simulink model "Simulation"  (R2023b)
settings: Solver=FixedStepAuto  StartTime=0  StopTime=H  FixedStep=fixed_step_size  RelTol=1e-3
values from neighbouring files (symbols this model uses):
  a_p = load_pu(:,3)    [Matlab_1_Generate_Case_Params.m]
  a_q = load_pu(:,6)    [Matlab_1_Generate_Case_Params.m]
  b_p = load_pu(:,4)    [Matlab_1_Generate_Case_Params.m]
  b_q = load_pu(:,7)    [Matlab_1_Generate_Case_Params.m]
  Be = zeros(Nn,Ne)    [Matlab_1_Generate_Case_Params.m]
  Bibr = zeros(Nn,Nibr)    [Matlab_1_Generate_Case_Params.m]
  Bload = zeros(Nn,Nload)    [Matlab_1_Generate_Case_Params.m]
  Bsh = zeros(Nn,Nsh)    [Matlab_1_Generate_Case_Params.m]
  C_f = gen_pu(:,7)    [Matlab_1_Generate_Case_Params.m]
  c_p = load_pu(:,5)    [Matlab_1_Generate_Case_Params.m]
  c_q = load_pu(:,8)    [Matlab_1_Generate_Case_Params.m]
  C_sh = busC(busC~=0)    [Matlab_1_Generate_Case_Params.m]
  Cdc = gen_pu(:,3)    [Matlab_1_Generate_Case_Params.m]
  f_b = 50    [Matlab_1_Generate_Case_Params.m]
  fixed_step_size = 1e-4    (= 0.0001)    [Matlab_2_Ref_Loop.m]
  ix_ibr_max = gen_pu(:,9) .* s_ibr_nom    [Matlab_1_Generate_Case_Params.m]
  jump_time = H/10    [Matlab_2_Ref_Loop.m]
  Kdc_I = omega_DC.^2 .* (Cdc./w_b) .* Vdc_n    [Matlab_1_Generate_Case_Params.m]
  Kdc_P = (2*gamma_DC.*omega_DC.*(Cdc./w_b).*Vdc_n + Pm_0./Vdc_n)    [Matlab_1_Generate_Case_Params.m]
  Ki_I = R_f./tau_CC    [Matlab_1_Generate_Case_Params.m]
  Ki_P = L_f./(w_b .* tau_CC)    [Matlab_1_Generate_Case_Params.m]
  Kpll_I = -omega_dPLL^2            *ones(Nibr,1)    [Matlab_1_Generate_Case_Params.m]
  Kpll_P = -2*gamma_dPLL*omega_dPLL *ones(Nibr,1)    [Matlab_1_Generate_Case_Params.m]
  Kpq_I = 1/tau_PQ      *ones(Nibr,1)    [Matlab_1_Generate_Case_Params.m]
  Kpq_P = tau_CC/tau_PQ *ones(Nibr,1)    [Matlab_1_Generate_Case_Params.m]
  Kv_I = zeros(Nibr,1)    [Matlab_1_Generate_Case_Params.m]
  Kv_P = C_f./(w_b*tau_VC)    [Matlab_1_Generate_Case_Params.m]
  L_f = gen_pu(:,6)    [Matlab_1_Generate_Case_Params.m]
  Le = br_pu(:,4)    [Matlab_1_Generate_Case_Params.m]
  Nibr = size(gen_pu,1)    [Matlab_1_Generate_Case_Params.m]
  R_f = gen_pu(:,5)    [Matlab_1_Generate_Case_Params.m]
  Re = br_pu(:,3)    [Matlab_1_Generate_Case_Params.m]
  ref_upd_time = ref_upd_time + jump_time    [Matlab_2_Ref_Loop.m]
  tau_dc = 5e-3 .* ones(Nibr,1)    [Matlab_1_Generate_Case_Params.m]
  tau_lpf_pll = ones(Nibr,1)/(2*pi*100)    [Matlab_1_Generate_Case_Params.m]
  Vdc_n = gen_pu(:,2)    [Matlab_1_Generate_Case_Params.m]
  w_0 = 1    [Matlab_1_Generate_Case_Params.m]
  w_b = 2*pi*f_b    (= 314.159265359)    [Matlab_1_Generate_Case_Params.m]
  w_c = 0.1 * w_b .* ones(Nibr,1)    [Matlab_1_Generate_Case_Params.m]
undefined symbols (not defined in the file or in its folder): hi_d_0, hi_q_0, hlpf_pll_0, hpll_0, hpq_d_0, hpq_q_0, hv_d_0, hv_q_0, hvdc_0, idc_0, ie_D_0, ie_Q_0, ix_d_0, ix_q_0, m_p_ibr_0, m_q_ibr_0, magnitude, n1_ratio, n2_ratio, p_ref_agc, p_ref_ed, Pload_fin, Pload_ini, q_ref_ed, Qload_fin, Qload_ini, score_0, theta_ibr_dq_0, vsh_D_0, vsh_Q_0, y_theta
libraries: spspowerguiLib x1
settings Model: Creator=tochoa  LastModifiedBy=tochoa
settings DataIOCC: InitialState=xFinal  SaveFormat=Array  SaveOutput=off  SaveState=on  DSMLogging=off

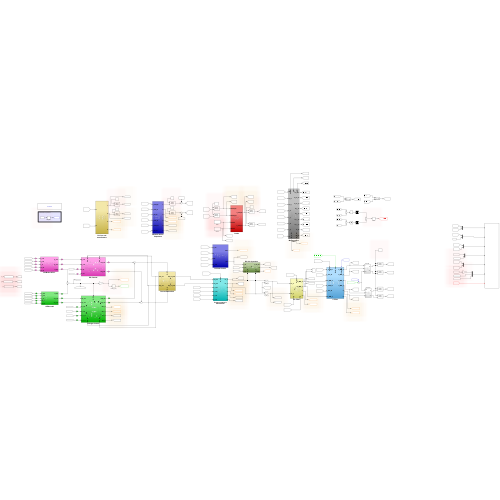
[thumbnail: Simulink's stored preview of the top-level diagram]
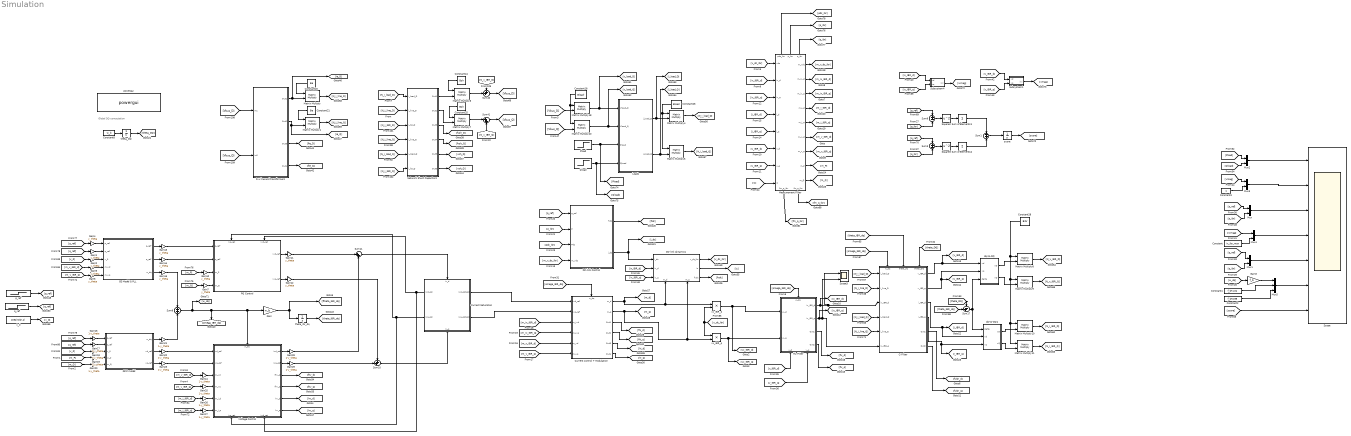
== system Simulation ==
  note: Global DQ computation
  C-Filter : Subsystem
      settings: PortSchema="{\"entries\":[{\"content\":{\"sides\":[{\"content\":{\"connectorIds\":[\"In1\",\"In2\",\"In3\",\"In4\",\"In5\",\"In6\"]},\"type\":\"ConnectorPlacement.EquallySpacedRectSide\",\"uuid\":\"8e2a7a25-a531-48a4-b0ad-05c1d749086a\"},{\"content\":{\"connectorIds\":[\"Out1\",\"Out2\",\"Out3\",\"Out4\",\"Out5\",\"Out6\"],\"side\":\"RIGHT\"},\"type\":\"ConnectorPlacement.EquallySpacedRectSide\",\"uuid\":\"d38f6705-4e72-49df-8302-a382bcc34c2b\"},{\"content\":{\"connectorIds\":[\"In7\",\"In8\",\"In9\"],\"side\":\"TOP\"},\"type\":\"ConnectorPlacement.EquallySpacedRectSide\",\"uuid\":\"5fb1126c-559e-482b-9e32-83c6aafed215\"}]},\"type\":\"ConnectorPlacement.EquallySpacedConnector\",\"uuid\":\"305c7e0f-6b62-4da7-9990-b58ec671b216\"}],\"packageUris\":[\"http://schema.mathworks.com/mf0/Connector/R2020b\"],\"version\":\"1.0\"}"
  Constant : Constant  Value=ix_ibr_max
  Constant1 : Constant  Value=f_b*1.01
  Constant18 : Constant  Value=Bload'  VectorParams1D=off
  Constant2 : Constant  Value=f_b*0.99
  Constant20 : Constant  Value=Be  VectorParams1D=off
  Constant21 : Constant  Value=Be  VectorParams1D=off
  Constant24 : Constant  Value=Bsh  VectorParams1D=off
  Constant25 : Constant  Value=Bsh  VectorParams1D=off
  Constant26 : Constant  Value=Bload  VectorParams1D=off
  Constant28 : Constant  Value=Bibr  VectorParams1D=off
  Constant3 : Constant
  Constant8 : Constant  Value=w_b  VectorParams1D=off
  Current Saturation : Subsystem
      settings: PortSchema="{\"entries\":[{\"content\":{\"sides\":[{\"content\":{\"connectorIds\":[\"Out3\",\"Out4\"]},\"type\":\"ConnectorPlacement.EquallySpacedRectSide\",\"uuid\":\"59f828dd-4cdf-4d05-93eb-9ca35b0898f6\"},{\"content\":{\"connectorIds\":[\"Out1\",\"Out2\"],\"side\":\"RIGHT\"},\"type\":\"ConnectorPlacement.EquallySpacedRectSide\",\"uuid\":\"2dafd29c-88ec-4fb5-8e24-68238ee40d02\"},{\"content\":{\"connectorIds\":[\"In1\"],\"side\":\"TOP\"},\"type\":\"ConnectorPlacement.EquallySpacedRectSide\",\"uuid\":\"d87b8d6c-f098-4820-b7b9-6c389e911afe\"},{\"content\":{\"connectorIds\":[\"In2\"],\"side\":\"BOTTOM\"},\"type\":\"ConnectorPlacement.EquallySpacedRectSide\",\"uuid\":\"42f80f0c-f330-4434-b01e-674189106f00\"}]},\"type\":\"ConnectorPlacement.EquallySpacedConnector\",\"uuid\":\"af101683-60bb-4d7f-95e3-aa4d232353b1\"}],\"packageUris\":[\"http://schema.mathworks.com/mf0/Connector/R2020b\"],\"version\":\"1.0\"}"
  Current control + Modulation : Subsystem
      settings: PortSchema="{\"entries\":[{\"content\":{\"sides\":[{\"content\":{\"connectorIds\":[\"In1\",\"In2\",\"In3\",\"In4\",\"In5\",\"In6\"]},\"type\":\"ConnectorPlacement.EquallySpacedRectSide\",\"uuid\":\"675af551-6b27-46ff-b785-f90e061c8dad\"},{\"content\":{\"connectorIds\":[\"Out1\",\"Out2\",\"Out3\",\"Out4\",\"Out5\",\"Out6\"],\"side\":\"RIGHT\"},\"type\":\"ConnectorPlacement.EquallySpacedRectSide\",\"uuid\":\"307b5813-d5df-486e-ab2e-3f3a32306549\"},{\"content\":{\"connectorIds\":[\"In7\"],\"side\":\"TOP\"},\"type\":\"ConnectorPlacement.EquallySpacedRectSide\",\"uuid\":\"c4e69032-edc2-40fd-8286-9db7cafe390c\"},{\"content\":{\"side\":\"BOTTOM\"},\"type\":\"ConnectorPlacement.EquallySpacedRectSide\",\"uuid\":\"6b3f8463-93c1-42af-a29a-0aa6610c4667\"}]},\"type\":\"ConnectorPlacement.EquallySpacedConnector\",\"uuid\":\"45ef52e4-2005-497d-a299-99787bf68448\"}],\"packageUris\":[\"http://schema.mathworks.com/mf0/Connector/R2020b\"],\"version\":\"1.0\"}"
  DC-link Control : Subsystem
  DC-link dynamics : Subsystem
      settings: PortSchema="{\"entries\":[{\"content\":{\"sides\":[{\"content\":{\"connectorIds\":[\"In1\",\"In2\",\"In3\"]},\"type\":\"ConnectorPlacement.EquallySpacedRectSide\",\"uuid\":\"447eb63a-0bf7-4feb-821b-73e5d968ae4d\"},{\"content\":{\"connectorIds\":[\"Out1\",\"Out2\",\"Out3\"],\"side\":\"RIGHT\"},\"type\":\"ConnectorPlacement.EquallySpacedRectSide\",\"uuid\":\"33bcdaf4-b7c0-46f4-89eb-0fbaf27441bb\"},{\"content\":{\"side\":\"TOP\"},\"type\":\"ConnectorPlacement.EquallySpacedRectSide\",\"uuid\":\"247e0d19-d01d-4c8d-8d8b-f925cd65c48b\"},{\"content\":{\"connectorIds\":[\"In4\",\"In5\"],\"side\":\"BOTTOM\"},\"type\":\"ConnectorPlacement.EquallySpacedRectSide\",\"uuid\":\"1c79db03-7d4d-4172-bf42-0a77b24cafad\"}]},\"type\":\"ConnectorPlacement.EquallySpacedConnector\",\"uuid\":\"95bb4a1b-05dc-4ef0-aadf-19065e959ee0\"}],\"packageUris\":[\"http://schema.mathworks.com/mf0/Connector/R2020b\"],\"version\":\"1.0\"}"
  GFM model : Subsystem
  GS Model & PLL : Subsystem
  Gain : Gain  Gain=w_b
  Gain{1..2,4..7,10..15} (12 alike) : Gain  Gain=y_theta
  Gain{16..29} (14 alike) : Gain  Gain=1-y_theta
  Gain3 : Gain  Gain=f_b
  Loads : Subsystem
  Matrix Multiply{,1,4..11,18,20} (12 alike) : Product  Multiplication=Matrix(*)
  Measurement Filter : Subsystem
      settings: PortSchema="{\"entries\":[{\"content\":{\"sides\":[{\"content\":{\"connectorIds\":[\"In1\",\"In2\",\"In3\",\"In4\",\"In5\",\"In6\",\"In7\",\"In8\"]},\"type\":\"ConnectorPlacement.EquallySpacedRectSide\",\"uuid\":\"98918fb3-b65c-4241-b442-bb1f5fea910b\"},{\"content\":{\"connectorIds\":[\"Out1\",\"Out2\",\"Out3\",\"Out4\",\"Out5\",\"Out6\",\"Out7\",\"Out8\",\"Out9\"],\"side\":\"RIGHT\"},\"type\":\"ConnectorPlacement.EquallySpacedRectSide\",\"uuid\":\"649fb4ae-e262-430c-9beb-89b7eebac1a9\"},{\"content\":{\"connectorIds\":[\"Out12\",\"Out13\",\"Out14\"],\"side\":\"TOP\"},\"type\":\"ConnectorPlacement.EquallySpacedRectSide\",\"uuid\":\"d52c67f5-4982-412d-bf56-15943d85a9e4\"},{\"content\":{\"connectorIds\":[\"Out10\",\"Out11\"],\"side\":\"BOTTOM\"},\"type\":\"ConnectorPlacement.EquallySpacedRectSide\",\"uuid\":\"595fde44-1ea5-4a4b-b726-c7089a857829\"}]},\"type\":\"ConnectorPlacement.EquallySpacedConnector\",\"uuid\":\"5996e241-2508-4a8a-a5c4-fe4266e8e1f1\"}],\"packageUris\":[\"http://schema.mathworks.com/mf0/Connector/R2020b\"],\"version\":\"1.0\"}"
  Mux{,1..4} (5 alike) : Mux  Inputs=2
  Mux5 : Mux  Inputs=3
  Network Shunt Capacitors : Subsystem
  PQ Control : Subsystem
      settings: PortSchema="{\"entries\":[{\"content\":{\"sides\":[{\"content\":{\"connectorIds\":[\"In1\",\"In2\",\"In3\",\"In4\"]},\"type\":\"ConnectorPlacement.EquallySpacedRectSide\",\"uuid\":\"6bcc99da-2192-4bac-b731-392b38773da6\"},{\"content\":{\"connectorIds\":[\"Out1\",\"Out2\"],\"side\":\"RIGHT\"},\"type\":\"ConnectorPlacement.EquallySpacedRectSide\",\"uuid\":\"3b353dec-d782-4d59-876f-75c55f7037f3\"},{\"content\":{\"connectorIds\":[\"In5\",\"In6\"],\"side\":\"TOP\"},\"type\":\"ConnectorPlacement.EquallySpacedRectSide\",\"uuid\":\"102326fa-9f47-43fa-b0a3-a887bb7894f3\"},{\"content\":{\"side\":\"BOTTOM\"},\"type\":\"ConnectorPlacement.EquallySpacedRectSide\",\"uuid\":\"2715e150-5598-4946-a5c2-168f1fe6a42a\"}]},\"type\":\"ConnectorPlacement.EquallySpacedConnector\",\"uuid\":\"24099521-315d-417b-ade6-b0d849696871\"}],\"packageUris\":[\"http://schema.mathworks.com/mf0/Connector/R2020b\"],\"version\":\"1.0\"}"
  Pload : Step  Time=jump_time  Before=double(Pload_ini)  After=double(Pload_fin)  SampleTime=0  VectorParams1D=off  ZeroCross=off
  Qload : Step  Time=jump_time  Before=double(Qload_ini)  After=double(Qload_fin)  SampleTime=0  VectorParams1D=off  ZeroCross=off
  R-L line and transformers : Subsystem
  RL-Filter : Subsystem
      settings: PortSchema="{\"entries\":[{\"content\":{\"sides\":[{\"content\":{\"connectorIds\":[\"In1\",\"In2\"]},\"type\":\"ConnectorPlacement.EquallySpacedRectSide\",\"uuid\":\"d1c64b46-6da4-4b5a-bbc1-7e56e3bdb69f\"},{\"content\":{\"connectorIds\":[\"Out1\",\"Out2\",\"Out3\",\"Out4\"],\"side\":\"RIGHT\"},\"type\":\"ConnectorPlacement.EquallySpacedRectSide\",\"uuid\":\"e46a9fd0-3779-4a4d-897e-928a7e15613b\"},{\"content\":{\"connectorIds\":[\"In3\"],\"side\":\"TOP\"},\"type\":\"ConnectorPlacement.EquallySpacedRectSide\",\"uuid\":\"7284c3ed-50d7-4bac-821c-918daee59977\"},{\"content\":{\"connectorIds\":[\"In4\",\"In5\"],\"side\":\"BOTTOM\"},\"type\":\"ConnectorPlacement.EquallySpacedRectSide\",\"uuid\":\"a4de9306-06dc-48a1-8948-b36bb4a619e3\"}]},\"type\":\"ConnectorPlacement.EquallySpacedConnector\",\"uuid\":\"1ec620e1-987b-4214-b86f-4b43fb0d2eea\"}],\"packageUris\":[\"http://schema.mathworks.com/mf0/Connector/R2020b\"],\"version\":\"1.0\"}"
  Scope : Scope  NumInputPorts=7
  Scope3 : Scope  NumInputPorts=2
  Square2 : Math  Operator=square
  Square3 : Math  Operator=square
  Subsystem1 : Subsystem
  Subsystem4 : Subsystem
  Sum of Elements1 : Sum  Inputs=+
  Sum of Elements2 : Sum  Inputs=+
  Sum1 : Sum  Inputs=+|+
  Sum10 : Sum  Inputs=++|
  Sum11 : Sum  Inputs=|++
  Sum17 : Sum  Inputs=-+|
  Sum3 : Sum  Inputs=+|-
  Sum40 : Sum  Inputs=++|
  Sum41 : Sum  Inputs=|++
  Sum8 : Sum  Inputs=+|+
  Sum9 : Sum  Inputs=+|-
  Voltage Control : Subsystem
      settings: PortSchema="{\"entries\":[{\"content\":{\"sides\":[{\"content\":{\"connectorIds\":[\"In1\",\"In2\",\"In3\",\"In4\",\"In5\",\"In6\"]},\"type\":\"ConnectorPlacement.EquallySpacedRectSide\",\"uuid\":\"20a64a1f-d721-4f6b-a097-588df04a85af\"},{\"content\":{\"connectorIds\":[\"Out1\",\"Out2\",\"Out3\",\"Out4\",\"Out5\",\"Out6\"],\"side\":\"RIGHT\"},\"type\":\"ConnectorPlacement.EquallySpacedRectSide\",\"uuid\":\"eabfc66f-1219-412f-8ead-b672ebf34355\"},{\"content\":{\"connectorIds\":[\"In7\"],\"side\":\"TOP\"},\"type\":\"ConnectorPlacement.EquallySpacedRectSide\",\"uuid\":\"5dffd779-7524-4ed4-b858-e78402c820de\"},{\"content\":{\"connectorIds\":[\"In8\",\"In9\"],\"side\":\"BOTTOM\"},\"type\":\"ConnectorPlacement.EquallySpacedRectSide\",\"uuid\":\"8d926eb8-5fba-49f0-a3b7-6537ca491f1b\"}]},\"type\":\"ConnectorPlacement.EquallySpacedConnector\",\"uuid\":\"c9bc2509-e264-46b8-8c5b-97763c943b87\"}],\"packageUris\":[\"http://schema.mathworks.com/mf0/Connector/R2020b\"],\"version\":\"1.0\"}"
  dq-to-DQ : Subsystem
  dq-to-DQ1 : Subsystem
  p_ref : Step  Time=ref_upd_time  Before=double(p_ref_ed)  After=double(p_ref_agc)  SampleTime=0  VectorParams1D=off  ZeroCross=off
  powergui : spspowerguiLib/powergui  Priority=1  SimulationMode=Continuous  SampleTime=fixed_step_size  frequency=50  Iterations=50  frequencyindice=0  Pbase=100e6  ErrMax=1e-4  UnitsV=kV  UnitsW=MW  buscounter=0  FunctionMessages=off  echomessages=off  EnableUseOfTLC=off  CurrentSourceSwitches=off  DisableSnubberDevices=off  DisableRonSwitches=off  DisableVfSwitches=off  DisplayEquations=off  AutomaticDiscreteSolvers=off  SolverType=Tustin/Backward Euler (TBE)  Interpol=off  ExternalGateDelay=off  methode=off  Ts=100  x0status=blocks  SPID=on  SwTol=0  HookPort=off  NonlinearTolerance=1e-4  nMaxIteration=100  ContinueOnMaxIteration=off  RestoreLinks=warning  ResistiveCurrentMeasurement=off  Frange=[0:2:500]  Ylog=off  Xlog=on  ShowGrid=off  save=off  variable=ZData  structure=0  ZoomFFT=off  StartTime=0.0  cycles=1  DisplayStyle=1  fundamental=60  FreqAxis=off  MaxFrequency=1000  frequencyindicesteady=1  RmsSteady=1  display=off
  q_ref : Step  Time=ref_upd_time  Before=double(q_ref_ed)  After=double(q_ref_ed)  SampleTime=0  VectorParams1D=off  ZeroCross=off
  score : Integrator  InitialCondition=score_0
  theta_DQ : Integrator
  theta_ibr_dq : Integrator  InitialCondition=theta_ibr_dq_0
  v_0 : Constant  Value=ones(Nibr,1)  VectorParams1D=off
  vx_IBR_d : Product
  vx_IBR_q : Product
  wires:
  theta_DQ/1 -> [theta_DQ]
  Constant8/1 -> theta_DQ/1
  R-L line and transformers/2(Out2) -> [ie_Q], Matrix Multiply1/2
  Matrix Multiply/1 -> [N_i_line_D]
  Constant20/1 -> Matrix Multiply/1
  R-L line and transformers/1(Out1) -> Matrix Multiply/2, [ie_D]
  Constant21/1 -> Matrix Multiply1/1
  Constant26/1 -> Matrix Multiply5/1, Matrix Multiply4/1
  Matrix Multiply5/1 -> [N_i_load_Q]
  Matrix Multiply4/1 -> [N_i_load_D]
  Matrix Multiply1/1 -> [N_i_line_Q]
  Pload/1 -> [Pload], Loads/3(Pload)
  Qload/1 -> [Qload], Loads/4(Qload)
  [N_i_load_D] -> Network Shunt Capacitors/1(i_load_D)
  [N_i_line_D] -> Network Shunt Capacitors/2(i_line_D)
  [N_i_IBR_D] -> Network Shunt Capacitors/3(i_ibr_D)
  [N_i_line_Q] -> Network Shunt Capacitors/4(i_line_Q)
  [N_i_load_Q] -> Network Shunt Capacitors/5(i_load_Q)
  [N_i_IBR_Q] -> Network Shunt Capacitors/6(i_ibr_Q)
  Constant24/1 -> Matrix Multiply6/1
  Matrix Multiply6/1 -> Sum40/2
  Network Shunt Capacitors/1(Out1) -> Matrix Multiply6/2
  Network Shunt Capacitors/2(Out2) -> Matrix Multiply7/2
  Matrix Multiply7/1 -> Sum41/1
  Constant25/1 -> Matrix Multiply7/1
  [N_v_IBR_D] -> Sum40/1
  [N_v_IBR_Q] -> Sum41/2
  Sum41/1 -> [Vbus_Q]
  Sum40/1 -> [Vbus_D]
  [Vbus_D] -> R-L line and transformers/1(In1)
  [Vbus_Q] -> R-L line and transformers/2(In6)
  DC-link dynamics/1(v_dc_ibr) -> [v_dc_ibr]
  [m_v_dc_ibr] -> DC-link Control/4(m_vdc)
  DC-link Control/2(i_dc) -> [i_dc], DC-link dynamics/1(i_dc)
  [v_dc_ibr] -> Measurement Filter/1(vdc)
  [ix_IBR_d] -> Measurement Filter/2(ix_d)
  [ix_IBR_q] -> Measurement Filter/3(ix_q)
  [i_IBR_d] -> Measurement Filter/4(i_d)
  [i_IBR_q] -> Measurement Filter/5(i_q)
  [v_IBR_d] -> Measurement Filter/6(v_d)
  [v_IBR_q] -> Measurement Filter/7(v_q)
  Measurement Filter/2(m_ix_d) -> [m_ix_IBR_d]
  Measurement Filter/3(m_ix_q) -> [m_ix_IBR_q]
  Measurement Filter/4(m_i_d) -> [m_i_IBR_d]
  Measurement Filter/5(m_i_q) -> [m_i_IBR_q]
  Measurement Filter/6(m_v_d) -> [m_v_IBR_d]
  Measurement Filter/7(m_v_q) -> [m_v_IBR_q]
  Measurement Filter/1(m_vdc) -> [m_v_dc_ibr]
  RL-Filter/1(ix_IBR_d) -> [ix_IBR_d], Scope3/1, C-Filter/3(ix_IBR_d)
  RL-Filter/2(ix_IBR_q) -> C-Filter/6(ix_IBR_q), Scope3/2, [ix_IBR_q]
  [m_v_IBR_d] -> Current control + Modulation/5(m_vd)
  [m_ix_IBR_d] -> Current control + Modulation/3(m_ixd)
  [m_ix_IBR_q] -> Current control + Modulation/4(m_ixq)
  [m_v_IBR_q] -> Current control + Modulation/6(m_vq)
  Measurement Filter/8(m_P) -> [m_P]
  Measurement Filter/9(m_Q) -> [m_Q]
  [omega_IBR_dq] -> RL-Filter/3(w_dq)
  [omega_IBR_dq] -> C-Filter/7(w_dq)
  [N_i_load_D] -> C-Filter/1(i_load_D)
  [N_i_line_D] -> C-Filter/2(i_line_D)
  [N_i_load_Q] -> C-Filter/4(i_load_Q)
  [N_i_line_Q] -> C-Filter/5(i_line_Q)
  [m_P] -> Gain19/1
  [m_Q] -> Gain20/1
  GFM model/2(vd_ref) -> Gain22/1
  [m_v_IBR_d] -> Gain24/1
  [m_v_IBR_q] -> Gain25/1
  Sum11/1 -> Current Saturation/1(ix_d)
  Sum10/1 -> Current Saturation/2(ix_q)
  [theta_DQ] -> C-Filter/9(theta_DQ)
  [theta_IBR_dq] -> C-Filter/8(theta_dq)
  [ix_IBR_d] -> DC-link dynamics/2(ix_d)
  [ix_IBR_q] -> DC-link dynamics/3(ix_q)
  vx_IBR_q/1 -> [vx_IBR_q], RL-Filter/2(vx_q)
  vx_IBR_d/1 -> RL-Filter/1(vx_d), [vx_IBR_d]
  dq-to-DQ1/2(xQ) -> Matrix Multiply11/2
  C-Filter/3(i_IBR_d) -> dq-to-DQ1/2(xd), [i_IBR_d]
  Matrix Multiply9/1 -> [N_v_IBR_Q]
  dq-to-DQ/2(xQ) -> Matrix Multiply9/2
  dq-to-DQ1/1(xD) -> Matrix Multiply10/2
  Matrix Multiply11/1 -> [N_i_IBR_Q]
  C-Filter/4(i_IBR_q) -> [i_IBR_q], dq-to-DQ1/3(xq)
  dq-to-DQ/1(xD) -> Matrix Multiply8/2
  Matrix Multiply8/1 -> [N_v_IBR_D]
  Constant28/1 -> Matrix Multiply9/1, Matrix Multiply10/1, Matrix Multiply11/1, Matrix Multiply8/1
  [theta_IBR_dq] -> Sum17/2
  [theta_DQ] -> Sum17/1
  Sum17/1 -> dq-to-DQ1/1(delta), dq-to-DQ/3(delta)
  Matrix Multiply10/1 -> [N_i_IBR_D]
  C-Filter/1(v_IBR_d) -> dq-to-DQ/1(xd), [v_IBR_d]
  C-Filter/2(v_IBR_q) -> dq-to-DQ/2(xq), [v_IBR_q]
  Sum8/1 -> [w_dq], Gain/1, Voltage Control/7(w_dq), [omega_IBR_dq]
  [v_IBR_d] -> RL-Filter/4(v_d)
  [v_IBR_q] -> RL-Filter/5(v_q)
  Constant18/1 -> Matrix Multiply20/1, Matrix Multiply18/1
  [Vbus_D] -> Matrix Multiply18/2
  [Vbus_Q] -> Matrix Multiply20/2
  Matrix Multiply20/1 -> [v_load_Q], Loads/2(Vload_Q)
  Loads/2(i_load_Q) -> [i_load_Q], Matrix Multiply5/2
  Loads/1(i_load_D) -> [i_load_D], Matrix Multiply4/2
  Matrix Multiply18/1 -> [v_load_D], Loads/1(Vload_D)
  GFM model/3(vq_ref) -> Gain23/1
  [m_i_IBR_d] -> Gain26/1
  [m_i_IBR_q] -> Gain27/1
  Gain/1 -> [ftheta_IBR_dq], theta_ibr_dq/1
  theta_ibr_dq/1 -> [theta_IBR_dq]
  DC-link dynamics/2(iz) -> [iz]
  [omega_IBR_dq] -> Current control + Modulation/7(w_dq)
  C-Filter/5(Out1) -> [fvibr_d]
  C-Filter/6(Out2) -> [fvibr_q]
  RL-Filter/3(Out1) -> [fix_d]
  RL-Filter/4(Out2) -> [fix_q]
  DC-link dynamics/3(fvdc) -> [fvdc]
  Current control + Modulation/3(Out1) -> [fhi_d]
  Current control + Modulation/4(Out2) -> [fhi_q]
  Voltage Control/3(fhv_d) -> [fhv_d]
  Voltage Control/4(fhv_q) -> [fhv_q]
  Network Shunt Capacitors/3(Out3) -> [fvsh_D]
  Network Shunt Capacitors/4(Out4) -> [fvsh_Q]
  R-L line and transformers/3(Out3) -> [fie_D]
  R-L line and transformers/4(Out4) -> [fie_Q]
  [v_dc_ibr] -> vx_IBR_d/2, vx_IBR_q/1
  Current control + Modulation/1(m_d) -> [m_d], DC-link dynamics/4(m_d), vx_IBR_d/1
  Current control + Modulation/2(m_q) -> DC-link dynamics/5(m_q), vx_IBR_q/2, [m_q]
  [iz] -> Measurement Filter/8(iz)
  Voltage Control/5(hv_d) -> [hv_d]
  Voltage Control/6(hv_q) -> [hv_q]
  Current control + Modulation/5(Out3) -> [hi_d]
  Current control + Modulation/6(Out4) -> [hi_q]
  Network Shunt Capacitors/5(Out5) -> [vsh_D]
  Network Shunt Capacitors/6(Out6) -> [vsh_Q]
  DC-link Control/1(fidc) -> [fidc]
  [p_ibr] -> Sum9/2
  Sum9/1 -> Square2/1
  Square2/1 -> Sum of Elements1/1
  p_ref/1 -> [p_ref]
  q_ref/1 -> [q_ref]
  v_0/1 -> [v_0]
  [q_ibr] -> Sum3/2
  Sum3/1 -> Square3/1
  Square3/1 -> Sum of Elements2/1
  [q_ref] -> Sum3/1
  [p_ref] -> Sum9/1
  [m_v_IBR_q] -> Gain6/1
  [p_ref] -> Gain16/1
  [q_ref] -> Gain17/1
  [v_0] -> Gain18/1
  GFM model/1(w_dq) -> Gain21/1
  Voltage Control/2(ixq_ref) -> Gain29/1
  Voltage Control/1(ixd_ref) -> Gain28/1
  PQ Control/2(ixq_ref) -> Gain12/1
  PQ Control/1(ixd_ref) -> Gain11/1
  [m_P] -> Gain10/1
  [m_Q] -> Gain7/1
  Current Saturation/2(ixq_ref_sat) -> Current control + Modulation/2(ixq_ref)
  Current Saturation/1(ixd_ref_sat) -> Current control + Modulation/1(ixd_ref)
  Current Saturation/3(ixd_ret) -> PQ Control/6(ixd_ret), Voltage Control/9(ixd_ret)
  Current Saturation/4(ixq_ret) -> Voltage Control/8(ixq_ret), PQ Control/5(ixq_ret)
  GS Model & PLL/1(p_ref') -> Gain13/1
  GS Model & PLL/2(q_ref') -> Gain14/1
  GS Model & PLL/3(w_dq) -> Gain15/1
  [p_ref] -> Gain4/1
  [q_ref] -> Gain1/1
  [v_0] -> Gain2/1
  [m_v_IBR_d] -> Gain5/1
  Gain4/1 -> GS Model & PLL/1(p_ref)
  Gain1/1 -> GS Model & PLL/2(q_ref)
  Gain2/1 -> GS Model & PLL/3(v_0)
  Gain5/1 -> GS Model & PLL/4(m_vd)
  Gain6/1 -> GS Model & PLL/5(m_vq)
  Gain10/1 -> PQ Control/3(m_P)
  Gain7/1 -> PQ Control/4(m_Q)
  Gain11/1 -> Sum11/1
  Gain12/1 -> Sum10/1
  Gain13/1 -> PQ Control/1(p_ref')
  Gain14/1 -> PQ Control/2(q_ref')
  Gain15/1 -> Sum8/1
  Gain16/1 -> GFM model/1(p_ref)
  Gain17/1 -> GFM model/2(q_ref)
  Gain18/1 -> GFM model/3(v_0)
  Gain19/1 -> GFM model/4(m_P)
  Gain20/1 -> GFM model/5(m_Q)
  Gain21/1 -> Sum8/2
  Gain22/1 -> Voltage Control/1(vd_ref)
  Gain23/1 -> Voltage Control/2(vq_ref)
  Gain24/1 -> Voltage Control/3(m_vd)
  Gain25/1 -> Voltage Control/4(m_vq)
  Gain26/1 -> Voltage Control/5(m_i_d)
  Gain27/1 -> Voltage Control/6(m_i_q)
  Gain28/1 -> Sum11/2
  Gain29/1 -> Sum10/2
  [p_ref] -> DC-link Control/1(p_ref)
  [p_ibr] -> DC-link Control/2(P)
  [pdc_ibr] -> DC-link Control/3(Pdc)
  score/1 -> [score]
  Measurement Filter/10(fm_p_ibr) -> [fm_p_ibr]
  Measurement Filter/11(fm_q_ibr) -> [fm_q_ibr]
  [ix_IBR_d] -> Subsystem4/1(xd)
  [ix_IBR_q] -> Subsystem4/2(xq)
  Subsystem4/1(|x|) -> [ixmag]
  Subsystem1/1(|x|) -> [vmag]
  [v_IBR_d] -> Subsystem1/1(xd)
  [v_IBR_q] -> Subsystem1/2(xq)
  [p_ref] -> Mux/1
  [p_ibr] -> Mux/2
  [q_ibr] -> Mux1/2
  [q_ref] -> Mux1/1
  Mux/1 -> Scope/3
  Mux1/1 -> Scope/5
  [w_dq] -> Gain3/1
  [ixmag] -> Mux4/1
  [vmag] -> Mux3/1
  [Pload] -> Mux2/1
  [Qload] -> Mux2/2
  Mux2/1 -> Scope/1
  [score] -> Scope/7
  Constant3/1 -> Mux3/2
  Mux3/1 -> Scope/2
  Constant/1 -> Mux4/2
  Mux4/1 -> Scope/4
  Gain3/1 -> Mux5/1
  Constant1/1 -> Mux5/2
  Constant2/1 -> Mux5/3
  Mux5/1 -> Scope/6
  Sum1/1 -> score/1
  Measurement Filter/13(p_ibr) -> [p_ibr]
  Measurement Filter/14(q_ibr) -> [q_ibr]
  Measurement Filter/12(pdc_ibr) -> [pdc_ibr]
  Sum of Elements1/1 -> Sum1/1
  Sum of Elements2/1 -> Sum1/2

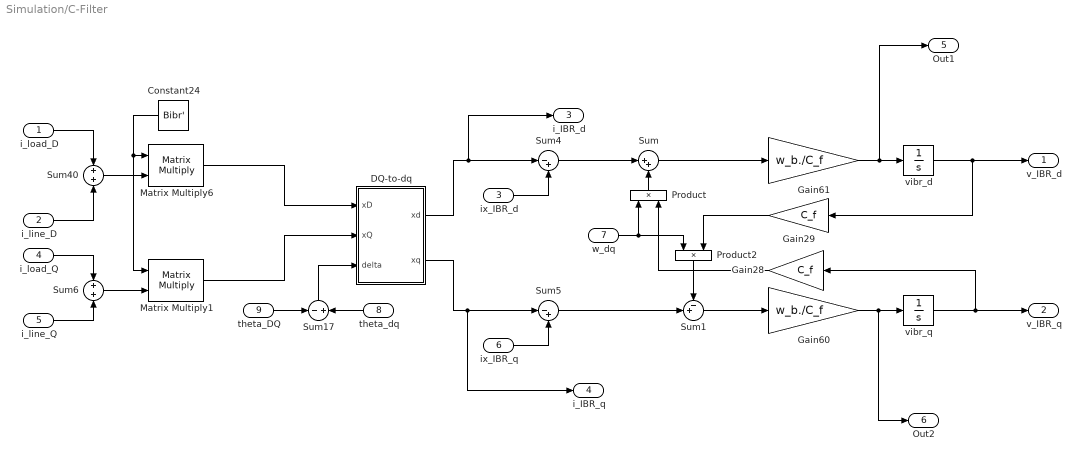
== system Simulation/C-Filter ==
  i_load_D : Inport
  i_line_D : Inport  Port=2
  ix_IBR_d : Inport  Port=3
  i_load_Q : Inport  Port=4
  i_line_Q : Inport  Port=5
  ix_IBR_q : Inport  Port=6
  w_dq : Inport  Port=7
  theta_dq : Inport  Port=8
  theta_DQ : Inport  Port=9
  Constant24 : Constant  Value=Bibr'  VectorParams1D=off
  DQ-to-dq : Subsystem
  Gain28 : Gain  Gain=C_f
  Gain29 : Gain  Gain=C_f
  Gain60 : Gain  Gain=w_b./C_f
  Gain61 : Gain  Gain=w_b./C_f
  Matrix Multiply1 : Product  Multiplication=Matrix(*)
  Matrix Multiply6 : Product  Multiplication=Matrix(*)
  Product : Product
  Product2 : Product
  Sum : Sum  Inputs=|++
  Sum1 : Sum  Inputs=-+|
  Sum17 : Sum  Inputs=-|+
  Sum4 : Sum  Inputs=|-+
  Sum40 : Sum
  Sum5 : Sum  Inputs=|-+
  Sum6 : Sum
  vibr_d : Integrator  InitialCondition=ones(Nibr,1)
  vibr_q : Integrator  InitialCondition=zeros(Nibr,1)
  v_IBR_d : Outport
  v_IBR_q : Outport  Port=2
  i_IBR_d : Outport  Port=3
  i_IBR_q : Outport  Port=4
  Out1 : Outport  Port=5
  Out2 : Outport  Port=6
  wires:
  Sum1/1 -> Gain60/1
  Gain29/1 -> Product2/2
  Product/1 -> Sum/2
  ix_IBR_q/1 -> Sum5/2
  Sum/1 -> Gain61/1
  Sum4/1 -> Sum/1
  Sum5/1 -> Sum1/2
  Gain61/1 -> Out1/1, vibr_d/1
  Gain60/1 -> Out2/1, vibr_q/1
  Matrix Multiply6/1 -> DQ-to-dq/1(xD)
  Sum40/1 -> Matrix Multiply6/2
  Constant24/1 -> Matrix Multiply1/1, Matrix Multiply6/1
  i_line_D/1 -> Sum40/2
  ix_IBR_d/1 -> Sum4/2
  i_load_D/1 -> Sum40/1
  Matrix Multiply1/1 -> DQ-to-dq/2(xQ)
  Sum6/1 -> Matrix Multiply1/2
  i_load_Q/1 -> Sum6/1
  i_line_Q/1 -> Sum6/2
  vibr_d/1 -> Gain29/1, v_IBR_d/1
  vibr_q/1 -> v_IBR_q/1, Gain28/1
  theta_DQ/1 -> Sum17/1
  Sum17/1 -> DQ-to-dq/3(delta)
  theta_dq/1 -> Sum17/2
  Gain28/1 -> Product/2
  Product2/1 -> Sum1/1
  w_dq/1 -> Product2/1, Product/1
  DQ-to-dq/1(xd) -> i_IBR_d/1, Sum4/1
  DQ-to-dq/2(xq) -> i_IBR_q/1, Sum5/1

== system Simulation/Current Saturation ==
  ix_d : Inport
  ix_q : Inport  Port=2
  Constant1 : Constant  Value=ix_ibr_max
  Divide2 : Product  Inputs=*/
  Product2 : Product
  Product3 : Product
  Saturation : Saturate  UpperLimit=1  LowerLimit=0
  Subsystem4 : Subsystem
  Sum5 : Sum  Inputs=-|+
  Sum8 : Sum  Inputs=-|+
  ixd_ref_sat : Outport
  ixq_ref_sat : Outport  Port=2
  ixd_ret : Outport  Port=3
  ixq_ret : Outport  Port=4
  wires:
  ix_q/1 -> Product3/2, Sum8/1, Subsystem4/2(xq)
  Subsystem4/1(|x|) -> Divide2/2
  Product2/1 -> ixd_ref_sat/1, Sum5/2
  Product3/1 -> ixq_ref_sat/1, Sum8/2
  ix_d/1 -> Product2/1, Sum5/1, Subsystem4/1(xd)
  Constant1/1 -> Divide2/1
  Sum5/1 -> ixd_ret/1
  Sum8/1 -> ixq_ret/1
  Saturation/1 -> Product2/2, Product3/1
  Divide2/1 -> Saturation/1

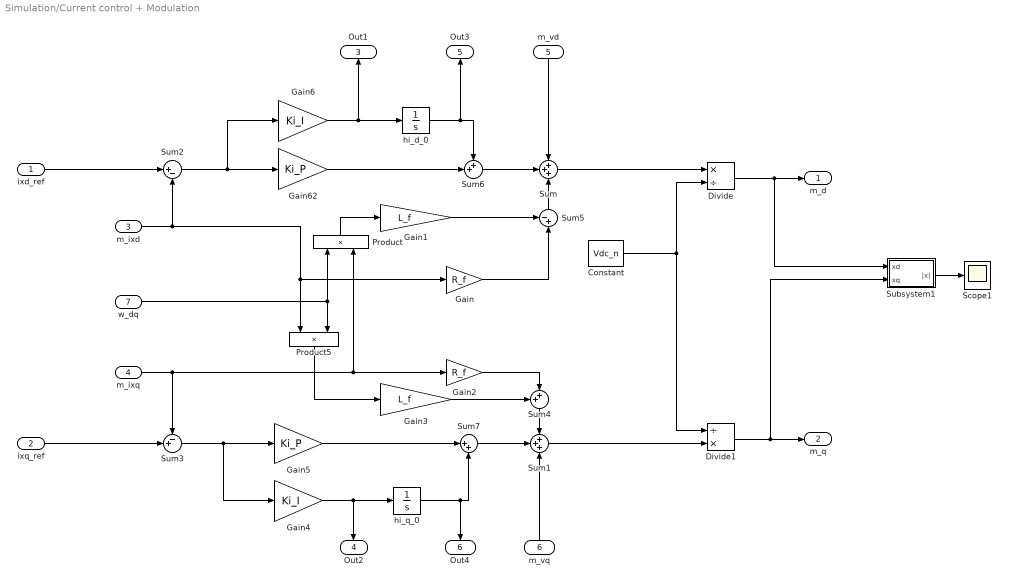
== system Simulation/Current control + Modulation ==
  ixd_ref : Inport
  ixq_ref : Inport  Port=2
  m_ixd : Inport  Port=3
  m_ixq : Inport  Port=4
  m_vd : Inport  Port=5
  m_vq : Inport  Port=6
  w_dq : Inport  Port=7
  Constant : Constant  Value=Vdc_n
  Divide : Product  Inputs=*/
  Divide1 : Product  Inputs=/*
  Gain : Gain  Gain=R_f
  Gain1 : Gain  Gain=L_f
  Gain2 : Gain  Gain=R_f
  Gain3 : Gain  Gain=L_f
  Gain4 : Gain  Gain=Ki_I
  Gain5 : Gain  Gain=Ki_P
  Gain6 : Gain  Gain=Ki_I
  Gain62 : Gain  Gain=Ki_P
  Product : Product
  Product5 : Product
  Scope1 : Scope
  Subsystem1 : Subsystem
  Sum : Sum  Inputs=+++
  Sum1 : Sum  Inputs=+++
  Sum2 : Sum  Inputs=|+-
  Sum3 : Sum  Inputs=-+|
  Sum4 : Sum  Inputs=++|
  Sum5 : Sum  Inputs=-+|
  Sum6 : Sum  Inputs=++|
  Sum7 : Sum  Inputs=|++
  hi_d_0 : Integrator  InitialCondition=hi_d_0
  hi_q_0 : Integrator  InitialCondition=hi_q_0
  m_d : Outport
  m_q : Outport  Port=2
  Out1 : Outport  Port=3
  Out2 : Outport  Port=4
  Out3 : Outport  Port=5
  Out4 : Outport  Port=6
  wires:
  Gain62/1 -> Sum6/2
  Gain3/1 -> Sum4/1
  Gain5/1 -> Sum7/1
  Sum6/1 -> Sum/2
  Gain2/1 -> Sum4/2
  Sum5/1 -> Sum/3
  m_ixq/1 -> Gain2/1, Product/2, Sum3/1
  Sum7/1 -> Sum1/2
  m_vd/1 -> Sum/1
  Sum4/1 -> Sum1/1
  Gain/1 -> Sum5/2
  Gain1/1 -> Sum5/1
  m_vq/1 -> Sum1/3
  Product/1 -> Gain1/1
  Product5/1 -> Gain3/1
  w_dq/1 -> Product/1, Product5/2
  m_ixd/1 -> Gain/1, Product5/1, Sum2/2
  Sum/1 -> Divide/1
  Sum2/1 -> Gain62/1, Gain6/1
  hi_q_0/1 -> Sum7/2, Out4/1
  hi_d_0/1 -> Sum6/1, Out3/1
  Sum3/1 -> Gain5/1, Gain4/1
  Constant/1 -> Divide1/1, Divide/2
  Sum1/1 -> Divide1/2
  Divide/1 -> Subsystem1/1(xd), m_d/1
  Divide1/1 -> Subsystem1/2(xq), m_q/1
  Subsystem1/1(|x|) -> Scope1/1
  ixd_ref/1 -> Sum2/1
  ixq_ref/1 -> Sum3/2
  Gain6/1 -> hi_d_0/1, Out1/1
  Gain4/1 -> hi_q_0/1, Out2/1

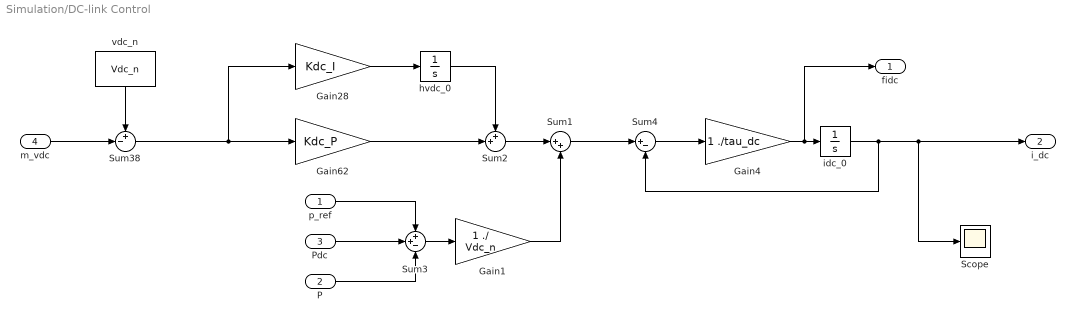
== system Simulation/DC-link Control ==
  p_ref : Inport
  P : Inport  Port=2
  Pdc : Inport  Port=3
  m_vdc : Inport  Port=4
  Gain1 : Gain  Gain=1 ./ Vdc_n
  Gain28 : Gain  Gain=Kdc_I
  Gain4 : Gain  Gain=1 ./tau_dc
  Gain62 : Gain  Gain=Kdc_P
  Scope : Scope
  Sum1 : Sum  Inputs=|++
  Sum2 : Sum  Inputs=++|
  Sum3 : Sum  Inputs=++-
  Sum38 : Sum  Inputs=+-|
  Sum4 : Sum  Inputs=|+-
  hvdc_0 : Integrator  InitialCondition=hvdc_0
  idc_0 : Integrator  InitialCondition=idc_0
  vdc_n : Constant  Value=Vdc_n
  fidc : Outport
  i_dc : Outport  Port=2
  wires:
  Gain62/1 -> Sum2/2
  vdc_n/1 -> Sum38/1
  m_vdc/1 -> Sum38/2
  idc_0/1 -> Sum4/2, Scope/1, i_dc/1
  Sum4/1 -> Gain4/1
  Gain4/1 -> fidc/1, idc_0/1
  Sum2/1 -> Sum1/1
  Gain28/1 -> hvdc_0/1
  Sum38/1 -> Gain62/1, Gain28/1
  hvdc_0/1 -> Sum2/1
  Sum1/1 -> Sum4/1
  Gain1/1 -> Sum1/2
  P/1 -> Sum3/3
  Pdc/1 -> Sum3/2
  p_ref/1 -> Sum3/1
  Sum3/1 -> Gain1/1

== system Simulation/DC-link dynamics ==
  i_dc : Inport
  ix_d : Inport  Port=2
  ix_q : Inport  Port=3
  m_d : Inport  Port=4
  m_q : Inport  Port=5
  Gain58 : Gain  Gain=w_b./Cdc
  Product10 : Product
  Product5 : Product
  Sum39 : Sum  Inputs=-|+
  i : Sum  Inputs=+|+
  vdc : Integrator  InitialCondition=Vdc_n
  v_dc_ibr : Outport
  iz : Outport  Port=2
  fvdc : Outport  Port=3
  wires:
  Product10/1 -> i/1
  vdc/1 -> v_dc_ibr/1
  ix_q/1 -> Product10/2
  ix_d/1 -> Product5/2
  Gain58/1 -> fvdc/1, vdc/1
  Product5/1 -> i/2
  m_q/1 -> Product10/1
  m_d/1 -> Product5/1
  Sum39/1 -> Gain58/1
  i_dc/1 -> Sum39/2
  i/1 -> iz/1, Sum39/1

== system Simulation/GFM model ==
  p_ref : Inport
  q_ref : Inport  Port=2
  v_0 : Inport  Port=3
  m_P : Inport  Port=4
  m_Q : Inport  Port=5
  Constant1 : Constant  Value=w_0  VectorParams1D=off
  Gain2 : Gain  Gain=n2_ratio
  Gain28 : Gain  Gain=n1_ratio
  Sum1 : Sum  Inputs=|+-
  Sum2 : Sum  Inputs=-+|
  Sum3 : Sum  Inputs=|++
  Sum4 : Sum  Inputs=|++
  v_q_ref_is_zero : Constant  Value=zeros(Nibr,1)  VectorParams1D=off
  w_dq : Outport
  vd_ref : Outport  Port=2
  vq_ref : Outport  Port=3
  wires:
  Sum1/1 -> Gain28/1
  m_P/1 -> Sum1/2
  p_ref/1 -> Sum1/1
  v_0/1 -> Sum3/2
  v_q_ref_is_zero/1 -> vq_ref/1
  Constant1/1 -> Sum4/1
  Gain28/1 -> Sum4/2
  m_Q/1 -> Sum2/1
  q_ref/1 -> Sum2/2
  Sum2/1 -> Gain2/1
  Gain2/1 -> Sum3/1
  Sum3/1 -> vd_ref/1
  Sum4/1 -> w_dq/1

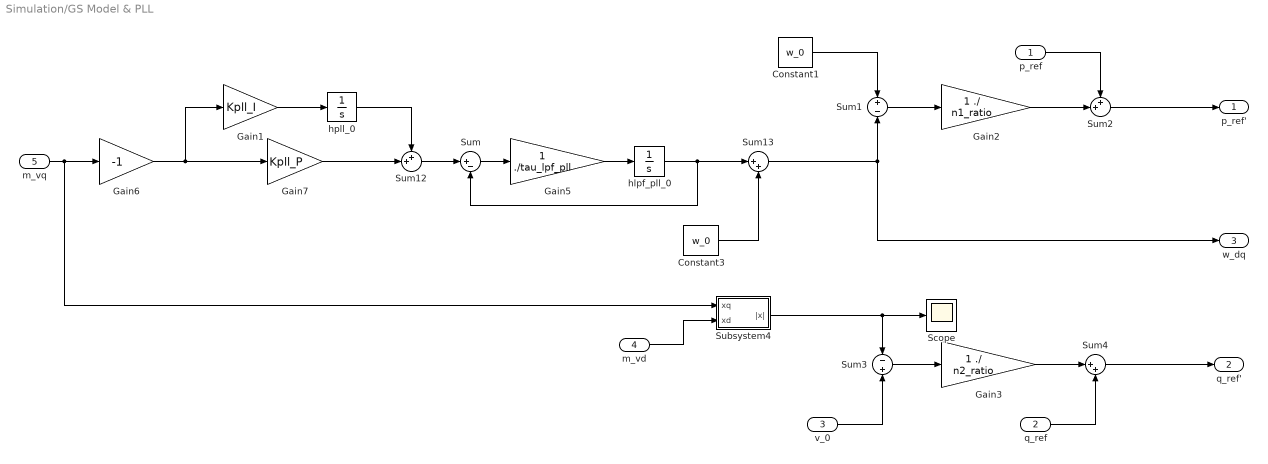
== system Simulation/GS Model & PLL ==
  p_ref : Inport
  q_ref : Inport  Port=2
  v_0 : Inport  Port=3
  m_vd : Inport  Port=4
  m_vq : Inport  Port=5
  Constant1 : Constant  Value=w_0  VectorParams1D=off
  Constant3 : Constant  Value=w_0  VectorParams1D=off
  Gain1 : Gain  Gain=Kpll_I
  Gain2 : Gain  Gain=1 ./ n1_ratio
  Gain3 : Gain  Gain=1 ./ n2_ratio
  Gain5 : Gain  Gain=1 ./tau_lpf_pll
  Gain6 : Gain  Gain=-1
  Gain7 : Gain  Gain=Kpll_P
  Scope : Scope
  Subsystem4 : Subsystem
  Sum : Sum  Inputs=|+-
  Sum1 : Sum  Inputs=+|-
  Sum12 : Sum  Inputs=++|
  Sum13 : Sum  Inputs=|++
  Sum2 : Sum  Inputs=++|
  Sum3 : Sum  Inputs=-|+
  Sum4 : Sum  Inputs=|++
  hlpf_pll_0 : Integrator  InitialCondition=hlpf_pll_0
  hpll_0 : Integrator  InitialCondition=hpll_0
  p_ref' : Outport
  q_ref' : Outport  Port=2
  w_dq : Outport  Port=3
  wires:
  Gain7/1 -> Sum12/2
  hpll_0/1 -> Sum12/1
  Constant3/1 -> Sum13/2
  Gain1/1 -> hpll_0/1
  m_vq/1 -> Subsystem4/1(xq), Gain6/1
  Gain6/1 -> Gain1/1, Gain7/1
  Constant1/1 -> Sum1/1
  Sum1/1 -> Gain2/1
  Gain2/1 -> Sum2/2
  p_ref/1 -> Sum2/1
  Sum2/1 -> p_ref'/1
  m_vd/1 -> Subsystem4/2(xd)
  v_0/1 -> Sum3/2
  Sum3/1 -> Gain3/1
  Gain3/1 -> Sum4/1
  q_ref/1 -> Sum4/2
  Sum4/1 -> q_ref'/1
  Sum/1 -> Gain5/1
  Sum12/1 -> Sum/1
  hlpf_pll_0/1 -> Sum/2, Sum13/1
  Gain5/1 -> hlpf_pll_0/1
  Sum13/1 -> Sum1/2, w_dq/1
  Subsystem4/1(|x|) -> Scope/1, Sum3/1

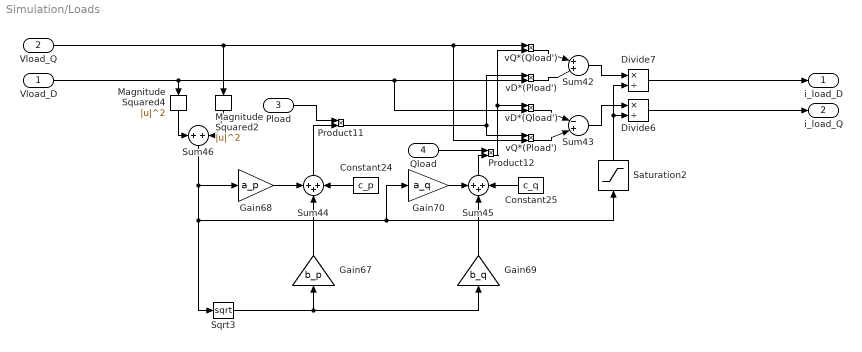
== system Simulation/Loads ==
  Vload_D : Inport
  Vload_Q : Inport  Port=2
  Pload : Inport  Port=3
  Qload : Inport  Port=4
  Constant24 : Constant  Value=c_p
  Constant25 : Constant  Value=c_q
  Divide6 : Product  Inputs=*/
  Divide7 : Product  Inputs=*/
  Gain67 : Gain  Gain=b_p
  Gain68 : Gain  Gain=a_p
  Gain69 : Gain  Gain=b_q
  Gain70 : Gain  Gain=a_q
  Magnitude Squared2 : Math  Operator=magnitude^2
  Magnitude Squared4 : Math  Operator=magnitude^2
  Product11 : Product
  Product12 : Product
  Saturation2 : Saturate  UpperLimit=inf  LowerLimit=1e-5  ZeroCross=off
  Sqrt3 : Sqrt
  Sum42 : Sum  Inputs=|++|
  Sum43 : Sum  Inputs=|-+|
  Sum44 : Sum  Inputs=+++
  Sum45 : Sum  Inputs=+++
  Sum46 : Sum  InputSameDT=on  SaturateOnIntegerOverflow=on  OutDataTypeStr=Inherit: Same as first input
  vD*(Pload') : Product
  vD*(Qload') : Product
  vQ*(Pload') : Product
  vQ*(Qload') : Product
  i_load_D : Outport
  i_load_Q : Outport  Port=2
  wires:
  Saturation2/1 -> Divide7/2, Divide6/2
  Gain68/1 -> Sum44/1
  Sum46/1 -> Sqrt3/1, Saturation2/1, Gain70/1, Gain68/1
  Product12/1 -> vQ*(Qload')/2, vD*(Qload')/1
  vQ*(Qload')/1 -> Sum42/1
  Constant25/1 -> Sum45/3
  Gain70/1 -> Sum45/1
  Gain67/1 -> Sum44/2
  vD*(Pload')/1 -> Sum42/2
  Magnitude Squared2/1 -> Sum46/2
  Magnitude Squared4/1 -> Sum46/1
  Product11/1 -> vD*(Pload')/1, vQ*(Pload')/1
  vQ*(Pload')/1 -> Sum43/2
  Pload/1 -> Product11/1
  vD*(Qload')/1 -> Sum43/1
  Divide7/1 -> i_load_D/1
  Constant24/1 -> Sum44/3
  Gain69/1 -> Sum45/2
  Sum43/1 -> Divide6/1
  Sum44/1 -> Product11/2
  Divide6/1 -> i_load_Q/1
  Sum45/1 -> Product12/2
  Sqrt3/1 -> Gain69/1, Gain67/1
  Sum42/1 -> Divide7/1
  Qload/1 -> Product12/1
  Vload_Q/1 -> vQ*(Pload')/2, vQ*(Qload')/1, Magnitude Squared2/1
  Vload_D/1 -> vD*(Pload')/2, vD*(Qload')/2, Magnitude Squared4/1

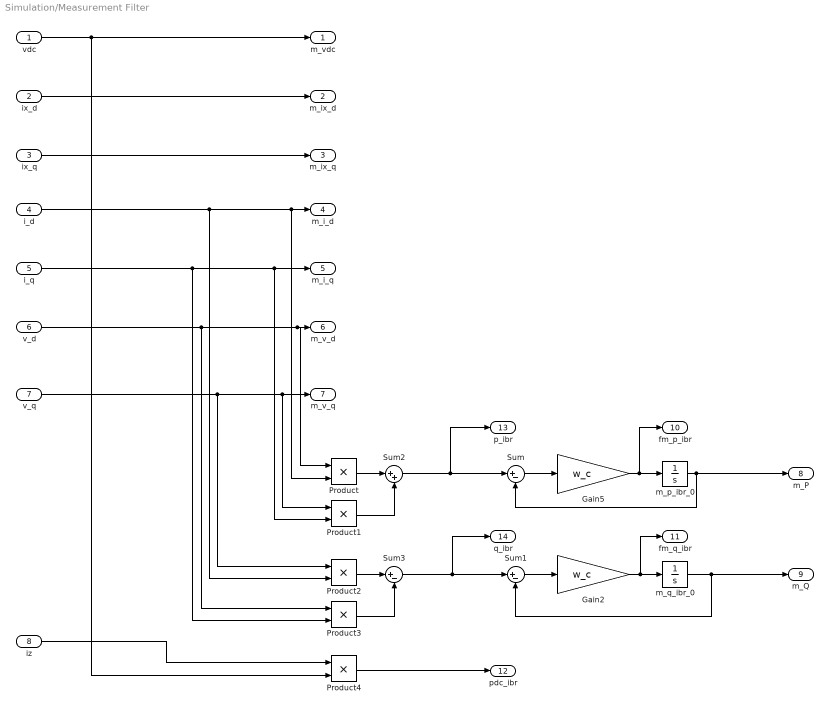
== system Simulation/Measurement Filter ==
  vdc : Inport
  ix_d : Inport  Port=2
  ix_q : Inport  Port=3
  i_d : Inport  Port=4
  i_q : Inport  Port=5
  v_d : Inport  Port=6
  v_q : Inport  Port=7
  iz : Inport  Port=8
  Gain2 : Gain  Gain=w_c
  Gain5 : Gain  Gain=w_c
  Product{,1..4} (5 alike) : Product
  Sum : Sum  Inputs=|+-
  Sum1 : Sum  Inputs=|+-
  Sum2 : Sum  Inputs=|++
  Sum3 : Sum  Inputs=|+-
  m_p_ibr_0 : Integrator  InitialCondition=m_p_ibr_0
  m_q_ibr_0 : Integrator  InitialCondition=m_q_ibr_0
  m_vdc : Outport
  m_ix_d : Outport  Port=2
  m_ix_q : Outport  Port=3
  m_i_d : Outport  Port=4
  m_i_q : Outport  Port=5
  m_v_d : Outport  Port=6
  m_v_q : Outport  Port=7
  m_P : Outport  Port=8
  m_Q : Outport  Port=9
  fm_p_ibr : Outport  Port=10
  fm_q_ibr : Outport  Port=11
  pdc_ibr : Outport  Port=12
  p_ibr : Outport  Port=13
  q_ibr : Outport  Port=14
  wires:
  i_d/1 -> Product/2, m_i_d/1, Product2/2
  ix_d/1 -> m_ix_d/1
  Product/1 -> Sum2/1
  Product1/1 -> Sum2/2
  Product3/1 -> Sum3/2
  Product2/1 -> Sum3/1
  ix_q/1 -> m_ix_q/1
  i_q/1 -> Product1/2, m_i_q/1, Product3/2
  v_d/1 -> Product/1, m_v_d/1, Product3/1
  v_q/1 -> m_v_q/1, Product1/1, Product2/1
  Sum/1 -> Gain5/1
  Sum2/1 -> p_ibr/1, Sum/1
  Sum1/1 -> Gain2/1
  Sum3/1 -> q_ibr/1, Sum1/1
  m_p_ibr_0/1 -> Sum/2, m_P/1
  m_q_ibr_0/1 -> Sum1/2, m_Q/1
  iz/1 -> Product4/1
  vdc/1 -> m_vdc/1, Product4/2
  Gain5/1 -> fm_p_ibr/1, m_p_ibr_0/1
  Gain2/1 -> fm_q_ibr/1, m_q_ibr_0/1
  Product4/1 -> pdc_ibr/1

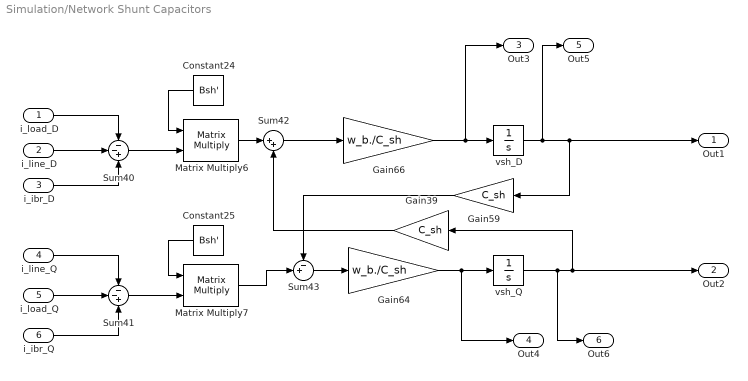
== system Simulation/Network Shunt Capacitors ==
  i_load_D : Inport
  i_line_D : Inport  Port=2
  i_ibr_D : Inport  Port=3
  i_line_Q : Inport  Port=4
  i_load_Q : Inport  Port=5
  i_ibr_Q : Inport  Port=6
  Constant24 : Constant  Value=Bsh'  VectorParams1D=off
  Constant25 : Constant  Value=Bsh'  VectorParams1D=off
  Gain39 : Gain  Gain=C_sh
  Gain59 : Gain  Gain=C_sh
  Gain64 : Gain  Gain=w_b./C_sh
  Gain66 : Gain  Gain=w_b./C_sh
  Matrix Multiply6 : Product  Multiplication=Matrix(*)
  Matrix Multiply7 : Product  Multiplication=Matrix(*)
  Sum40 : Sum  Inputs=--+
  Sum41 : Sum  Inputs=--+
  Sum42 : Sum  Inputs=|++
  Sum43 : Sum  Inputs=-+|
  vsh_D : Integrator  InitialCondition=vsh_D_0
  vsh_Q : Integrator  InitialCondition=vsh_Q_0
  Out1 : Outport
  Out2 : Outport  Port=2
  Out3 : Outport  Port=3
  Out4 : Outport  Port=4
  Out5 : Outport  Port=5
  Out6 : Outport  Port=6
  wires:
  Gain64/1 -> Out4/1, vsh_Q/1
  Constant25/1 -> Matrix Multiply7/1
  Gain66/1 -> Out3/1, vsh_D/1
  Sum43/1 -> Gain64/1
  i_load_D/1 -> Sum40/1
  vsh_Q/1 -> Out6/1, Out2/1, Gain39/1
  Constant24/1 -> Matrix Multiply6/1
  Sum42/1 -> Gain66/1
  i_line_D/1 -> Sum40/2
  vsh_D/1 -> Out5/1, Out1/1, Gain59/1
  Matrix Multiply7/1 -> Sum43/2
  Gain39/1 -> Sum42/2
  Sum40/1 -> Matrix Multiply6/2
  Gain59/1 -> Sum43/1
  Matrix Multiply6/1 -> Sum42/1
  Sum41/1 -> Matrix Multiply7/2
  i_load_Q/1 -> Sum41/2
  i_line_Q/1 -> Sum41/1
  i_ibr_D/1 -> Sum40/3
  i_ibr_Q/1 -> Sum41/3

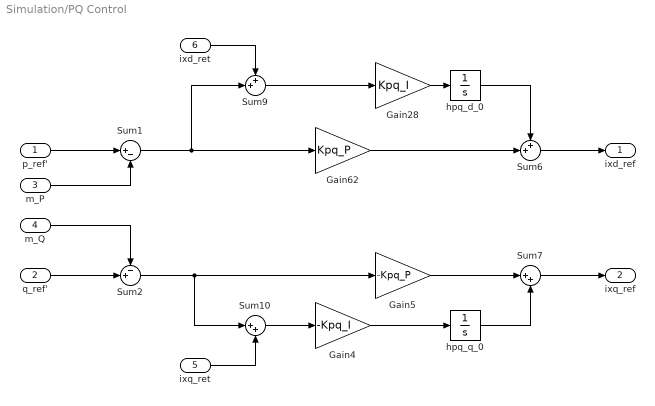
== system Simulation/PQ Control ==
  p_ref' : Inport
  q_ref' : Inport  Port=2
  m_P : Inport  Port=3
  m_Q : Inport  Port=4
  ixq_ret : Inport  Port=5
  ixd_ret : Inport  Port=6
  Gain28 : Gain  Gain=Kpq_I
  Gain4 : Gain  Gain=-Kpq_I
  Gain5 : Gain  Gain=-Kpq_P
  Gain62 : Gain  Gain=Kpq_P
  Sum1 : Sum  Inputs=|+-
  Sum10 : Sum  Inputs=|++
  Sum2 : Sum  Inputs=-+|
  Sum6 : Sum  Inputs=++|
  Sum7 : Sum  Inputs=|++
  Sum9 : Sum  Inputs=++|
  hpq_d_0 : Integrator  InitialCondition=hpq_d_0
  hpq_q_0 : Integrator  InitialCondition=hpq_q_0
  ixd_ref : Outport
  ixq_ref : Outport  Port=2
  wires:
  Sum1/1 -> Sum9/2, Gain62/1
  Sum2/1 -> Sum10/1, Gain5/1
  m_P/1 -> Sum1/2
  m_Q/1 -> Sum2/1
  p_ref'/1 -> Sum1/1
  q_ref'/1 -> Sum2/2
  hpq_d_0/1 -> Sum6/1
  Gain62/1 -> Sum6/2
  Gain28/1 -> hpq_d_0/1
  Gain4/1 -> hpq_q_0/1
  hpq_q_0/1 -> Sum7/2
  Gain5/1 -> Sum7/1
  Sum9/1 -> Gain28/1
  Sum10/1 -> Gain4/1
  ixd_ret/1 -> Sum9/1
  ixq_ret/1 -> Sum10/2
  Sum7/1 -> ixq_ref/1
  Sum6/1 -> ixd_ref/1

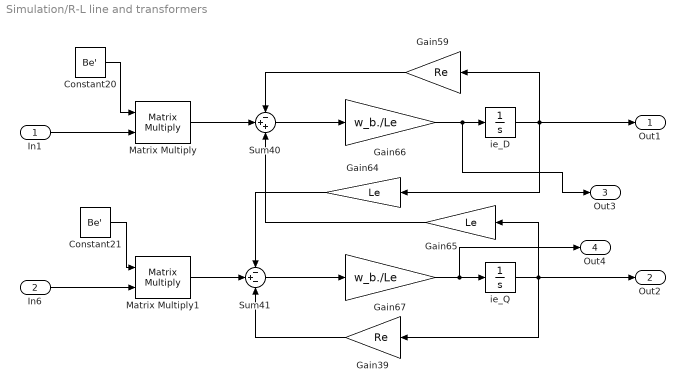
== system Simulation/R-L line and transformers ==
  In1 : Inport
  In6 : Inport  Port=2
  Constant20 : Constant  Value=Be'  VectorParams1D=off
  Constant21 : Constant  Value=Be'  VectorParams1D=off
  Gain39 : Gain  Gain=Re
  Gain59 : Gain  Gain=Re
  Gain64 : Gain  Gain=Le
  Gain65 : Gain  Gain=Le
  Gain66 : Gain  Gain=w_b./Le
  Gain67 : Gain  Gain=w_b./Le
  Matrix Multiply : Product  Multiplication=Matrix(*)
  Matrix Multiply1 : Product  Multiplication=Matrix(*)
  Sum40 : Sum  Inputs=-++
  Sum41 : Sum  Inputs=-+-
  ie_D : Integrator  InitialCondition=ie_D_0
  ie_Q : Integrator  InitialCondition=ie_Q_0
  Out1 : Outport
  Out2 : Outport  Port=2
  Out3 : Outport  Port=3
  Out4 : Outport  Port=4
  wires:
  Constant21/1 -> Matrix Multiply1/1
  In6/1 -> Matrix Multiply1/2
  Gain65/1 -> Sum40/3
  Gain59/1 -> Sum40/1
  Matrix Multiply1/1 -> Sum41/2
  ie_Q/1 -> Out2/1, Gain39/1, Gain65/1
  Gain66/1 -> Out3/1, ie_D/1
  ie_D/1 -> Out1/1, Gain59/1, Gain64/1
  Gain39/1 -> Sum41/3
  Matrix Multiply/1 -> Sum40/2
  Constant20/1 -> Matrix Multiply/1
  Gain67/1 -> Out4/1, ie_Q/1
  Gain64/1 -> Sum41/1
  Sum41/1 -> Gain67/1
  Sum40/1 -> Gain66/1
  In1/1 -> Matrix Multiply/2

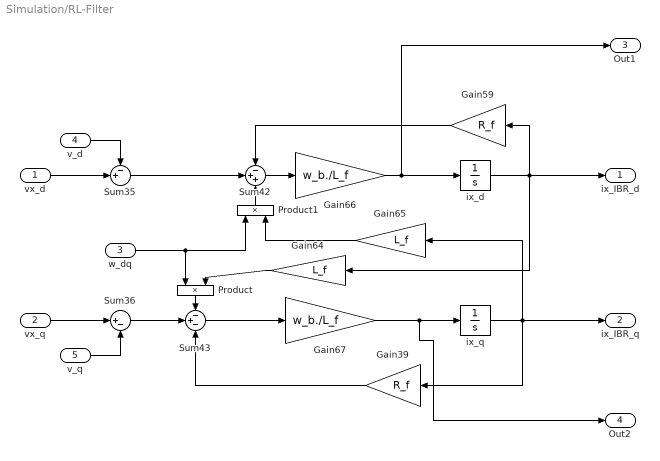
== system Simulation/RL-Filter ==
  vx_d : Inport
  vx_q : Inport  Port=2
  w_dq : Inport  Port=3
  v_d : Inport  Port=4
  v_q : Inport  Port=5
  Gain39 : Gain  Gain=R_f
  Gain59 : Gain  Gain=R_f
  Gain64 : Gain  Gain=L_f
  Gain65 : Gain  Gain=L_f
  Gain66 : Gain  Gain=w_b./L_f
  Gain67 : Gain  Gain=w_b./L_f
  Product : Product
  Product1 : Product
  Sum35 : Sum  Inputs=-+|
  Sum36 : Sum  Inputs=|+-
  Sum42 : Sum  Inputs=-++
  Sum43 : Sum  Inputs=-+-
  ix_d : Integrator  InitialCondition=ix_d_0
  ix_q : Integrator  InitialCondition=ix_q_0
  ix_IBR_d : Outport
  ix_IBR_q : Outport  Port=2
  Out1 : Outport  Port=3
  Out2 : Outport  Port=4
  wires:
  Gain59/1 -> Sum42/1
  Sum42/1 -> Gain66/1
  vx_q/1 -> Sum36/1
  vx_d/1 -> Sum35/2
  Sum43/1 -> Gain67/1
  Gain65/1 -> Product1/2
  Gain39/1 -> Sum43/3
  Gain64/1 -> Product/2
  Gain66/1 -> Out1/1, ix_d/1
  Gain67/1 -> Out2/1, ix_q/1
  ix_d/1 -> Gain64/1, Gain59/1, ix_IBR_d/1
  ix_q/1 -> ix_IBR_q/1, Gain39/1, Gain65/1
  Product/1 -> Sum43/1
  Product1/1 -> Sum42/3
  w_dq/1 -> Product1/1, Product/1
  v_q/1 -> Sum36/2
  v_d/1 -> Sum35/1
  Sum35/1 -> Sum42/2
  Sum36/1 -> Sum43/2

== system Simulation/Subsystem1 ==
  xd : Inport
  xq : Inport  Port=2
  Product : Product
  Product1 : Product
  Sqrt : Sqrt
  Sum4 : Sum
  |x| : Outport
  wires:
  Sqrt/1 -> |x|/1
  xd/1 -> Product/2, Product/1
  Product1/1 -> Sum4/2
  Product/1 -> Sum4/1
  xq/1 -> Product1/1, Product1/2
  Sum4/1 -> Sqrt/1

== system Simulation/Subsystem4 ==
  xd : Inport
  xq : Inport  Port=2
  Product : Product
  Product1 : Product
  Sqrt : Sqrt
  Sum4 : Sum
  |x| : Outport
  wires:
  Sqrt/1 -> |x|/1
  xd/1 -> Product/2, Product/1
  Product1/1 -> Sum4/2
  Product/1 -> Sum4/1
  xq/1 -> Product1/1, Product1/2
  Sum4/1 -> Sqrt/1

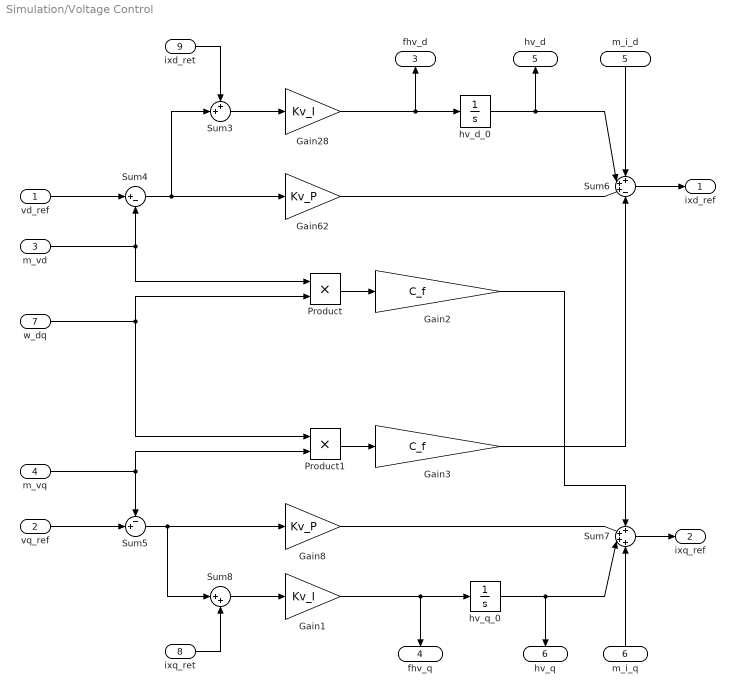
== system Simulation/Voltage Control ==
  vd_ref : Inport
  vq_ref : Inport  Port=2
  m_vd : Inport  Port=3
  m_vq : Inport  Port=4
  m_i_d : Inport  Port=5
  m_i_q : Inport  Port=6
  w_dq : Inport  Port=7
  ixq_ret : Inport  Port=8
  ixd_ret : Inport  Port=9
  Gain1 : Gain  Gain=Kv_I
  Gain2 : Gain  Gain=C_f
  Gain28 : Gain  Gain=Kv_I
  Gain3 : Gain  Gain=C_f
  Gain62 : Gain  Gain=Kv_P
  Gain8 : Gain  Gain=Kv_P
  Product : Product
  Product1 : Product
  Sum3 : Sum  Inputs=++|
  Sum4 : Sum  Inputs=|+-
  Sum5 : Sum  Inputs=-+|
  Sum6 : Sum  Inputs=+++-
  Sum7 : Sum  Inputs=++++
  Sum8 : Sum  Inputs=|++
  hv_d_0 : Integrator  InitialCondition=hv_d_0
  hv_q_0 : Integrator  InitialCondition=hv_q_0
  ixd_ref : Outport
  ixq_ref : Outport  Port=2
  fhv_d : Outport  Port=3
  fhv_q : Outport  Port=4
  hv_d : Outport  Port=5
  hv_q : Outport  Port=6
  wires:
  Gain62/1 -> Sum6/3
  Gain8/1 -> Sum7/2
  m_vd/1 -> Sum4/2, Product/1
  m_vq/1 -> Sum5/1, Product1/2
  w_dq/1 -> Product/2, Product1/1
  Product/1 -> Gain2/1
  Gain2/1 -> Sum7/1
  Product1/1 -> Gain3/1
  Gain3/1 -> Sum6/4
  m_i_d/1 -> Sum6/1
  m_i_q/1 -> Sum7/4
  Sum4/1 -> Sum3/2, Gain62/1
  vd_ref/1 -> Sum4/1
  vq_ref/1 -> Sum5/2
  Sum5/1 -> Sum8/1, Gain8/1
  hv_q_0/1 -> hv_q/1, Sum7/3
  Gain28/1 -> fhv_d/1, hv_d_0/1
  Gain1/1 -> hv_q_0/1, fhv_q/1
  hv_d_0/1 -> hv_d/1, Sum6/2
  Sum3/1 -> Gain28/1
  Sum8/1 -> Gain1/1
  Sum6/1 -> ixd_ref/1
  Sum7/1 -> ixq_ref/1
  ixd_ret/1 -> Sum3/1
  ixq_ret/1 -> Sum8/2

== system Simulation/dq-to-DQ ==
  xd : Inport
  xq : Inport  Port=2
  delta : Inport  Port=3
  Gain : Gain
  Sum6 : Sum  Inputs=|+-
  Sum8 : Sum  Inputs=|++
  Trigonometric Function : Trigonometry  Operator=cos  NumberOfIterations=121  OutputSignalType=real
  Trigonometric Function1 : Trigonometry  NumberOfIterations=121  OutputSignalType=real
  xd*cosd : Product
  xd*sind : Product
  xq*cosd : Product
  xq*sind : Product
  xD : Outport
  xQ : Outport  Port=2
  wires:
  xd*sind/1 -> Sum8/1
  Trigonometric Function/1 -> xq*cosd/2, xd*cosd/2
  xq*sind/1 -> Sum6/2
  xq*cosd/1 -> Sum8/2
  Trigonometric Function1/1 -> xq*sind/2, xd*sind/2
  Gain/1 -> Trigonometric Function1/1, Trigonometric Function/1
  xd/1 -> xd*cosd/1, xd*sind/1
  xq/1 -> xq*cosd/1, xq*sind/1
  xd*cosd/1 -> Sum6/1
  delta/1 -> Gain/1
  Sum6/1 -> xD/1
  Sum8/1 -> xQ/1

== system Simulation/dq-to-DQ1 ==
  delta : Inport
  xd : Inport  Port=2
  xq : Inport  Port=3
  Gain : Gain
  Sum6 : Sum  Inputs=|+-
  Sum8 : Sum  Inputs=|++
  Trigonometric Function : Trigonometry  Operator=cos  NumberOfIterations=121  OutputSignalType=real
  Trigonometric Function1 : Trigonometry  NumberOfIterations=121  OutputSignalType=real
  xd*cosd : Product
  xd*sind : Product
  xq*cosd : Product
  xq*sind : Product
  xD : Outport
  xQ : Outport  Port=2
  wires:
  xd*sind/1 -> Sum8/1
  Trigonometric Function/1 -> xq*cosd/2, xd*cosd/2
  xq*sind/1 -> Sum6/2
  xq*cosd/1 -> Sum8/2
  Trigonometric Function1/1 -> xq*sind/2, xd*sind/2
  Gain/1 -> Trigonometric Function1/1, Trigonometric Function/1
  xd/1 -> xd*cosd/1, xd*sind/1
  xq/1 -> xq*cosd/1, xq*sind/1
  xd*cosd/1 -> Sum6/1
  delta/1 -> Gain/1
  Sum6/1 -> xD/1
  Sum8/1 -> xQ/1

== system Simulation/C-Filter/DQ-to-dq ==
  xD : Inport
  xQ : Inport  Port=2
  delta : Inport  Port=3
  Gain : Gain  Gain=-1
  Sum6 : Sum  Inputs=|+-
  Sum8 : Sum  Inputs=|++
  Trigonometric Function : Trigonometry  Operator=cos  NumberOfIterations=121  OutputSignalType=real
  Trigonometric Function1 : Trigonometry  NumberOfIterations=121  OutputSignalType=real
  xD*cos(-d) : Product
  xD*sin(-d) : Product
  xQ*cos(-d) : Product
  xQ*sin(-d) : Product
  xd : Outport
  xq : Outport  Port=2
  wires:
  xD*sin(-d)/1 -> Sum8/1
  Trigonometric Function/1 -> xQ*cos(-d)/2, xD*cos(-d)/2
  xQ*sin(-d)/1 -> Sum6/2
  xQ*cos(-d)/1 -> Sum8/2
  Trigonometric Function1/1 -> xQ*sin(-d)/2, xD*sin(-d)/2
  Gain/1 -> Trigonometric Function1/1, Trigonometric Function/1
  xD/1 -> xD*cos(-d)/1, xD*sin(-d)/1
  xQ/1 -> xQ*cos(-d)/1, xQ*sin(-d)/1
  xD*cos(-d)/1 -> Sum6/1
  delta/1 -> Gain/1
  Sum6/1 -> xd/1
  Sum8/1 -> xq/1

== system Simulation/Current Saturation/Subsystem4 ==
  xd : Inport
  xq : Inport  Port=2
  Constant : Constant  Value=10^(-8)
  Product : Product
  Product1 : Product
  Sqrt : Sqrt
  Sum1 : Sum  Inputs=|++
  Sum4 : Sum
  |x| : Outport
  wires:
  Sqrt/1 -> |x|/1
  xd/1 -> Product/2, Product/1
  Product1/1 -> Sum4/2
  Product/1 -> Sum4/1
  xq/1 -> Product1/1, Product1/2
  Sum4/1 -> Sum1/1
  Sum1/1 -> Sqrt/1
  Constant/1 -> Sum1/2

== system Simulation/Current control + Modulation/Subsystem1 ==
  xd : Inport
  xq : Inport  Port=2
  Product : Product
  Product1 : Product
  Sqrt : Sqrt
  Sum4 : Sum
  |x| : Outport
  wires:
  Sqrt/1 -> |x|/1
  xd/1 -> Product/2, Product/1
  Product1/1 -> Sum4/2
  Sum4/1 -> Sqrt/1
  Product/1 -> Sum4/1
  xq/1 -> Product1/1, Product1/2

== system Simulation/GS Model & PLL/Subsystem4 ==
  xq : Inport
  xd : Inport  Port=2
  Product : Product
  Product1 : Product
  Sqrt : Sqrt
  Sum4 : Sum
  |x| : Outport
  wires:
  Sqrt/1 -> |x|/1
  xd/1 -> Product/2, Product/1
  Product1/1 -> Sum4/2
  Sum4/1 -> Sqrt/1
  Product/1 -> Sum4/1
  xq/1 -> Product1/1, Product1/2
